simulink model "buck_dcm_vs2_interval_flatten"  (Simulink 8.3)
settings: Solver=ode45  StartTime=0.0  StopTime=0.0375  RelTol=1e-3
settings Model: Creator=Luan Nguyen  LastModifiedBy=Luan Nguyen
settings DataIOCC: SignalLoggingSaveFormat=Dataset
settings DebuggingCC: UnderspecifiedInitializationDetection=Simplified  StateNameClashWarn=none
settings GRTTargetCC: CombineOutputUpdateFcns=on  GRTInterface=off

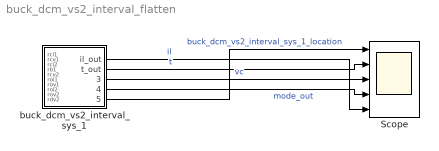
== system buck_dcm_vs2_interval_flatten ==
  Scope : Scope  NumInputPorts=5
      settings: YMin=-5~-5~-5~-5~-5  YMax=5~5~5~5~5  DataFormat=Structure
  buck_dcm_vs2_interval_sys_1 : Stateflow chart  TreatAsAtomicUnit=on
  wires:
  buck_dcm_vs2_interval_sys_1/5(buck_dcm_vs2_interval_sys_1_location) -> Scope/1  "buck_dcm_vs2_interval_sys_1_location"
  buck_dcm_vs2_interval_sys_1/2(t_out) -> Scope/2  "t"
  buck_dcm_vs2_interval_sys_1/3(vc_out) -> Scope/3  "vc"
  buck_dcm_vs2_interval_sys_1/4(mode_out_out) -> Scope/4  "mode_out"
  buck_dcm_vs2_interval_sys_1/1(il_out) -> Scope/5  "il"

== stateflow chart buck_dcm_vs2_interval_sys_1 ==
  settings: updateMethod=CONTINUOUS
  state charging_charging_controller
    du:
    il_dot = buckboost_template_1_a00c * il + rci1 + buckboost_template_1_a01c * vc + rcv1 + buckboost_template_1_b0c * Vs + rb1;
    vc_dot = buckboost_template_1_a10c * il + rci2 + buckboost_template_1_a11c * vc + rcv2 + buckboost_template_1_b1c * Vs;
    t_dot = 1;
    mode_out_dot = 0;
    il_out=il;
    t_out=t;
    vc_out=vc;
    mode_out_out=mode_out;
    buck_dcm_vs2_interval_sys_1_location =1;
  state discharging_discharging_controller
    du:
    il_dot = buckboost_template_1_a00o * il + roi1 + buckboost_template_1_a01o * vc + rov1 + buckboost_template_1_b0o * Vs;
    vc_dot = buckboost_template_1_a10o * il + roi2 + buckboost_template_1_a11o * vc + rov2 + buckboost_template_1_b1o * Vs;
    t_dot = 1;
    mode_out_dot = 0;
    il_out=il;
    t_out=t;
    vc_out=vc;
    mode_out_out=mode_out;
    buck_dcm_vs2_interval_sys_1_location =2;
  state dcm_discharging_controller
    du:
    il_dot = 0;
    vc_dot = buckboost_template_1_a11o * vc + rdv2 + buckboost_template_1_b1o * Vs;
    t_dot = 1;
    mode_out_dot = 0;
    il_out=il;
    t_out=t;
    vc_out=vc;
    mode_out_out=mode_out;
    buck_dcm_vs2_interval_sys_1_location =3;
  charging_charging_controller -> discharging_discharging_controller : [vc >= VcH]
      | {mode_out = 1;}
  discharging_discharging_controller -> dcm_discharging_controller [order 2] : [il <= 0 && vc > VcL]
  (default) -> charging_charging_controller : {il = 0;
      | vc = 0;
      | t = 0;
      | mode_out = 2;}
  discharging_discharging_controller -> charging_charging_controller [order 1] : [vc <= VcL]
      | {mode_out = 2;}
  dcm_discharging_controller -> charging_charging_controller : [vc <= VcL]
      | {mode_out = 2;}
  data: il_out output double; il local double; t_out output double; t local double; vc_out output double; vc local double; mode_out_out output double; mode_out local double; rci1 input double; rcv1 input double; rci2 input double; rb1 input double; rcv2 input double; roi1 input double; rov1 input double; roi2 input double; rov2 input double; rdv2 input double; buck_dcm_vs2_interval_sys_1_location output double; VcH constant double =12.1; buckboost_template_1_a11o constant double =-45.4545; tmax constant double =0.0375; buckboost_template_1_a01o constant double =-377.3585; VcL constant double =11.9; buckboost_template_1_a10o constant double =454.5455; Vs constant double =24; buckboost_template_1_a00o constant double =-196.2264; buckboost_template_1_b1o constant double =0; buckboost_template_1_b0o constant double =0; buckboost_template_1_a11c constant double =-45.4545; buckboost_template_1_b0c constant double =377.3585; buckboost_template_1_a10c constant double =454.5455; buckboost_template_1_b1c constant double =0; buckboost_template_1_bounds constant double =1000; buckboost_template_1_a01c constant double =-377.3585; buckboost_template_1_a00c constant double =-271.6981
  data il settings: updateMethod=SF_CONTINUOUS_TIME_DATA
  data t settings: updateMethod=SF_CONTINUOUS_TIME_DATA
  data vc settings: updateMethod=SF_CONTINUOUS_TIME_DATA
  data mode_out settings: updateMethod=SF_CONTINUOUS_TIME_DATA
  data rci1 settings: updateMethod=SF_CONTINUOUS_TIME_DATA
  data rcv1 settings: updateMethod=SF_CONTINUOUS_TIME_DATA
  data rci2 settings: updateMethod=SF_CONTINUOUS_TIME_DATA
  data rb1 settings: updateMethod=SF_CONTINUOUS_TIME_DATA
  data rcv2 settings: updateMethod=SF_CONTINUOUS_TIME_DATA
  data roi1 settings: updateMethod=SF_CONTINUOUS_TIME_DATA
  data rov1 settings: updateMethod=SF_CONTINUOUS_TIME_DATA
  data roi2 settings: updateMethod=SF_CONTINUOUS_TIME_DATA
  data rov2 settings: updateMethod=SF_CONTINUOUS_TIME_DATA
  data rdv2 settings: updateMethod=SF_CONTINUOUS_TIME_DATA
